simulink model "obwod_naprowadzania_JW"  (Simulink 10.2)
settings: Solver=VariableStepAuto  StartTime=0.0  StopTime=t_sim  MaxStep=0.005  EnableMultiTasking=on
values from neighbouring files (symbols this model uses):
  B_cel0 = deg2rad(-180)    [progaram_symulacyjny.m]
  E_cel0 = deg2rad(0)    [progaram_symulacyjny.m]
  v0 = 300    [progaram_symulacyjny.m]
  x0 = sqrt(23500^2-y0^2-z0^2)+v0*40    [progaram_symulacyjny.m]
  y0 = 0    [progaram_symulacyjny.m]
  z0 = 7000    [progaram_symulacyjny.m]
undefined symbols (not defined in the file or in its folder): beta_0_prim_srcp, caL, epsilon_0_prim_srcp, Fm, Fs, g, h_uwk, Im0, Im1, Is0, Is1, R, RB, RBC, RC, RE, REC, S, tm, ts, tster
libraries: simulink_extras x6, simulink x3
(part 1 of 2)
settings Model: Creator=Marcin  LastModifiedBy=rafal  SimulationMode=accelerator
settings SolverCC: AlgebraicLoopSolver=LineSearch
settings DataIOCC: SaveFormat=Dataset  SignalLoggingSaveFormat=Dataset  SaveOutput=off  SignalLogging=off  DSMLogging=off  SaveTime=off  ReturnWorkspaceOutputs=on  OutputOption=AdditionalOutputTimes  OutputTimes=[0 25]
settings OptimizationCC: BlockReduction=off  BooleanDataType=off  ExpressionDepthLimit=2147483647
settings DebuggingCC: AlgebraicLoopMsg=none  SaveWithParameterizedLinksMsg=none  SignalResolutionControl=TryResolveAllWithWarning  MultiTaskDSMMsg=warning  MultiTaskCondExecSysMsg=none  UnconnectedInputMsg=none  UnconnectedOutputMsg=none  StateNameClashWarn=warning
settings HardwareCC: TargetUnknown=on

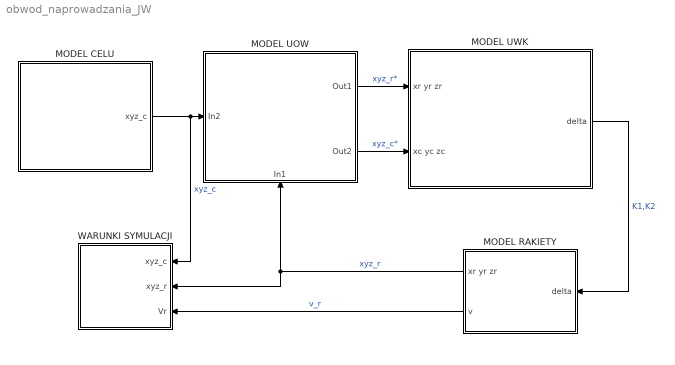
== system obwod_naprowadzania_JW ==
  MODEL CELU : Subsystem
      mask Display: image('C:\Users\rafal\Desktop\project inzynier\MATLAB\APP\photos\photo_target.jpg'); % Use "Edit Image" on toolstrip to change.
  MODEL RAKIETY : Subsystem
      mask Display: image('C:\Users\rafal\Desktop\project inzynier\MATLAB\APP\photos\photo_rocket.jpg'); % Use "Edit Image" on toolstrip to change.
  MODEL UOW : Subsystem
      settings: PortSchema="{\"entries\":[{\"content\":{\"sides\":[{\"content\":{\"connectorIds\":[\"In1\"]},\"type\":\"ConnectorPlacement.EquallySpacedRectSide\",\"uuid\":\"3befb01d-3bbd-4f2b-80c3-c30ac2a777af\"},{\"content\":{\"connectorIds\":[\"Out1\",\"Out2\"],\"side\":\"RIGHT\"},\"type\":\"ConnectorPlacement.EquallySpacedRectSide\",\"uuid\":\"03e5f92e-1691-4957-8f0b-6c1fa9d54603\"},{\"content\":{\"connectorIds\":[],\"side\":\"TOP\"},\"type\":\"ConnectorPlacement.EquallySpacedRectSide\",\"uuid\":\"07804cda-bb58-4fab-8fa4-61420b718606\"},{\"content\":{\"connectorIds\":[\"In2\"],\"side\":\"BOTTOM\"},\"type\":\"ConnectorPlacement.EquallySpacedRectSide\",\"uuid\":\"8550f404-f45b-4210-a410-eab1ae605921\"},{\"content\":{\"connectorIds\":[],\"side\":\"HIDDEN\"},\"type\":\"ConnectorPlacement.EquallySpacedRectSide\",\"uuid\":\"ae5e5650-e780-42f5-87a2-0961b270b42b\"}]},\"type\":\"ConnectorPlacement.EquallySpacedConnector\",\"uuid\":\"f3ed23f3-ebd5-40a8-abbc-f73b2ecd0d2f\"}],\"packageUris\":[\"http://schema.mathworks.com/mf0/Connector/R2020b\"],\"version\":\"1.0\"}"
      mask Display: image('C:\Users\rafal\Desktop\project inzynier\MATLAB\APP\photos\photo_radar.jpg'); % Use "Edit Image" on toolstrip to change.
  MODEL UWK : Subsystem
      mask Display: image('C:\Users\rafal\Desktop\project inzynier\MATLAB\APP\photos\photo_snr.jpg'); % Use "Edit Image" on toolstrip to change.
  WARUNKI SYMULACJI : Subsystem
  wires:
  MODEL UWK/1(delta) -> MODEL RAKIETY/1(delta)  "K1,K2"
  MODEL CELU/1(xyz_c) -> WARUNKI SYMULACJI/1(xyz_c), MODEL UOW/1(In2)  "xyz_c"
  MODEL RAKIETY/1(xr yr zr) -> WARUNKI SYMULACJI/2(xyz_r), MODEL UOW/2(In1)  "xyz_r"
  MODEL UOW/1(Out1) -> MODEL UWK/1(xr yr zr)  "xyz_r*"
  MODEL UOW/2(Out2) -> MODEL UWK/2(xc yc zc)  "xyz_c*"
  MODEL RAKIETY/2(v) -> WARUNKI SYMULACJI/3(Vr)  "v_r"

== system obwod_naprowadzania_JW/MODEL CELU ==
  Bus to Vector1 : BusToVector
  Model samolotu : Subsystem
  Wyliczanie przeciążeń : Subsystem
  Wyliczanie współrzędnych kartezjańskich samolotu : Subsystem
  xyz_c : Outport
  wires:
  Wyliczanie przeciążeń/1(n) -> [n]
  Model samolotu/1(y) -> Wyliczanie przeciążeń/1(In), Wyliczanie współrzędnych kartezjańskich samolotu/1(In)
  [n] -> Model samolotu/1(n)
  Wyliczanie współrzędnych kartezjańskich samolotu/1(xyz_c) -> Bus to Vector1/1
  Bus to Vector1/1 -> xyz_c/1

== system obwod_naprowadzania_JW/MODEL RAKIETY ==
  note: Px
  note: Pz
  note: Py
  note: M
  note: N
  delta : Inport
  10 rownan rozniczkowych : Subsystem
      mask Display: disp('Rownania rakiety')
  Bus Selector : BusSelector  OutputSignals=x_r,y_r,z_r,vr
  Demux : Demux  Outputs=10
      settings: DisplayOption=none
  Demux1 : Demux  Outputs=3
      settings: DisplayOption=none
  Funkcje w rownaniach rozniczkowych : Subsystem
      mask Display: disp('F(t), m(t), Iy(t), Iz(t)')
  Mux : Mux  Inputs=22
  Mux2 : Mux  Inputs=3
  One1 : Constant  OutDataTypeStr=Inherit: Inherit via back propagation
  Timer : Integrator
  To Workspace1 : ToWorkspace  VariableName=r_time  SampleTime=-1
      settings: MaxDataPoints=1
  Zaleznosci miedzy wprowadzonymi ukladami wspolrzednych : Subsystem
      mask Display: disp('mia, beta, alfa')
  Zaleznosci na skladowe sil i momentow aerodynamicznych : Subsystem
      mask Display: disp('Aero')
  "delta 1,2 -> delta m,n" : Subsystem  mask(Delta){}
      mask Display: disp('Delta')
  stala : Constant  Value=-1
  zg(t)*(-1) : Subsystem  mask(Dot Product){}
      mask help:
      | Inner (dot) product.
      | y=sum(u1.*u2)
      mask Help: Computes the inner (dot) product of the inputs: sum(u1.*u2).  The inputs are vectors of the same length. Output is a scalar.
      mask Display: disp('.\n')
  xr yr zr : Outport
  v : Outport  Port=2
  wires:
  Zaleznosci na skladowe sil i momentow aerodynamicznych/1(out_1) -> Mux/18
  Zaleznosci na skladowe sil i momentow aerodynamicznych/2(out_2) -> Mux/19
  Zaleznosci na skladowe sil i momentow aerodynamicznych/3(out_3) -> Mux/20
  Zaleznosci na skladowe sil i momentow aerodynamicznych/4(out_4) -> Mux/21
  Zaleznosci na skladowe sil i momentow aerodynamicznych/5(out_5) -> Mux/22
  Demux/1 -> Mux/1
  Demux/2 -> Mux/2
  Demux/3 -> Mux/3
  Demux/4 -> Mux/4
  Demux/5 -> Mux/5
  Demux/6 -> Mux/6
  Demux/8 -> Mux/8
  Demux/9 -> Mux/9
  Demux/10 -> Mux/10
  Demux/7 -> Mux/7
  Zaleznosci miedzy wprowadzonymi ukladami wspolrzednych/1(out_1) -> Mux/15
  Zaleznosci miedzy wprowadzonymi ukladami wspolrzednych/2(out_2) -> Mux/16, Zaleznosci na skladowe sil i momentow aerodynamicznych/1(beta)
  Zaleznosci miedzy wprowadzonymi ukladami wspolrzednych/3(out_3) -> Mux/17, Zaleznosci na skladowe sil i momentow aerodynamicznych/2(alfa)
  Bus Selector/1 -> Mux2/1  "<x_r>"
  Bus Selector/2 -> Mux2/2  "<y_r>"
  zg(t)*(-1)/1(out_1) -> Mux2/3
  Mux2/1 -> xr yr zr/1
  Demux1/1 -> Mux/11
  Demux1/2 -> Mux/12
  Demux1/3 -> Mux/13, Mux/14
  Funkcje w rownaniach rozniczkowych/1(out_1) -> Demux1/1
  Mux/1 -> 10 rownan rozniczkowych/1(in_1)
  10 rownan rozniczkowych/1(out_1) -> Bus Selector/1, Demux/1, Zaleznosci na skladowe sil i momentow aerodynamicznych/3(1-10), Zaleznosci miedzy wprowadzonymi ukladami wspolrzednych/1(in_1)
  delta/1 -> "delta 1,2 -> delta m,n"/1(delta_1,2)
  "delta 1,2 -> delta m,n"/1(delta_m,n) -> Zaleznosci na skladowe sil i momentow aerodynamicznych/4(delta)
  One1/1 -> Timer/1
  Timer/1 -> To Workspace1/1
  stala/1 -> zg(t)*(-1)/2(in_2)
  Bus Selector/3 -> zg(t)*(-1)/1(in_1)  "<z_r>"
  Bus Selector/4 -> v/1  "<vr>"

== system obwod_naprowadzania_JW/MODEL UOW ==
  In2 : Inport
  In1 : Inport  Port=2
  Cartesian to Spherical : simulink_extras/Transformations/Cartesian to Spherical
      settings: SourceProductBaseCode=SL
  Cartesian to Spherical1 : simulink_extras/Transformations/Cartesian to Spherical
      settings: SourceProductBaseCode=SL
  Demux3 : Demux  Outputs=3
      settings: DisplayOption=none
  Demux4 : Demux  Outputs=3
      settings: DisplayOption=none
  Mux : Mux  Inputs=3
  Mux1 : Mux  Inputs=3
  Spherical to Cartesian : simulink_extras/Transformations/Spherical to Cartesian
      settings: SourceProductBaseCode=SL
  Spherical to Cartesian1 : simulink_extras/Transformations/Spherical to Cartesian
      settings: SourceProductBaseCode=SL
  UOW C : Subsystem
  UOW R : Subsystem
  Out1 : Outport
  Out2 : Outport  Port=2
  wires:
  Demux4/3 -> Cartesian to Spherical/3
  In2/1 -> Demux4/1
  Cartesian to Spherical1/1 -> UOW R/1(R)
  Demux3/2 -> Cartesian to Spherical1/2
  Mux1/1 -> Out1/1
  Demux3/3 -> Cartesian to Spherical1/3
  Cartesian to Spherical/2 -> UOW C/2(B)
  Demux4/1 -> Cartesian to Spherical/1
  Demux3/1 -> Cartesian to Spherical1/1
  Demux4/2 -> Cartesian to Spherical/2
  Cartesian to Spherical/3 -> UOW C/3(E)
  Cartesian to Spherical/1 -> UOW C/1(R)
  Cartesian to Spherical1/2 -> UOW R/2(B)
  Cartesian to Spherical1/3 -> UOW R/3(E)
  In1/1 -> Demux3/1
  Mux/1 -> Out2/1
  UOW R/1(R*) -> Spherical to Cartesian/1
  UOW R/2(B*) -> Spherical to Cartesian/2
  UOW R/3(E*) -> Spherical to Cartesian/3
  Spherical to Cartesian/3 -> Mux1/3
  Spherical to Cartesian/2 -> Mux1/2
  Spherical to Cartesian/1 -> Mux1/1
  UOW C/2(B*) -> Spherical to Cartesian1/2
  UOW C/1(R*) -> Spherical to Cartesian1/1
  UOW C/3(E*) -> Spherical to Cartesian1/3
  Spherical to Cartesian1/3 -> Mux/3
  Spherical to Cartesian1/2 -> Mux/2
  Spherical to Cartesian1/1 -> Mux/1

== system obwod_naprowadzania_JW/MODEL UWK ==
  xr yr zr : Inport
  xc yc zc : Inport  Port=2
  Demux : Demux  Outputs=2
      settings: DisplayOption=none
  Demux1 : Demux  Outputs=2
      settings: DisplayOption=none
  "K -> delta" : Subsystem  mask(Delta){}
      mask Display: disp('Delta')
  Komendy Kierowania Waskie Pasmo : Subsystem  mask(Komendy){}
      mask Display: disp('K1, K2')
  Mux1 : Mux  Inputs=2
  Odchyki : Subsystem  mask(Mask){}
      mask Display: disp('h, fi_prim')
  Przelicznik TP : Subsystem  mask(TP){}
      mask Display: disp('TP')
  delta : Outport
  wires:
  Komendy Kierowania Waskie Pasmo/1(K1) -> "K -> delta"/1(K1)
  Komendy Kierowania Waskie Pasmo/2(K2) -> "K -> delta"/2(K2)
  Przelicznik TP/1(Out) -> Komendy Kierowania Waskie Pasmo/1(In1)
  "K -> delta"/1(delta1) -> Mux1/1
  "K -> delta"/2(delta2) -> Mux1/2
  Demux/1 -> Przelicznik TP/3(fi1c_prim)
  Demux/2 -> Przelicznik TP/4(fi2c_prim)
  Mux1/1 -> delta/1
  Demux1/2 -> Przelicznik TP/2(h2fi2)
  Demux1/1 -> Przelicznik TP/1(h1fi1)
  xr yr zr/1 -> Odchyki/1(xr yr zr)
  xc yc zc/1 -> Odchyki/2(xc yc zc)
  Odchyki/2(fi_prim) -> Demux/1
  Odchyki/1(h) -> Demux1/1
  Odchyki/3(gammaR) -> Komendy Kierowania Waskie Pasmo/2(gammaR)

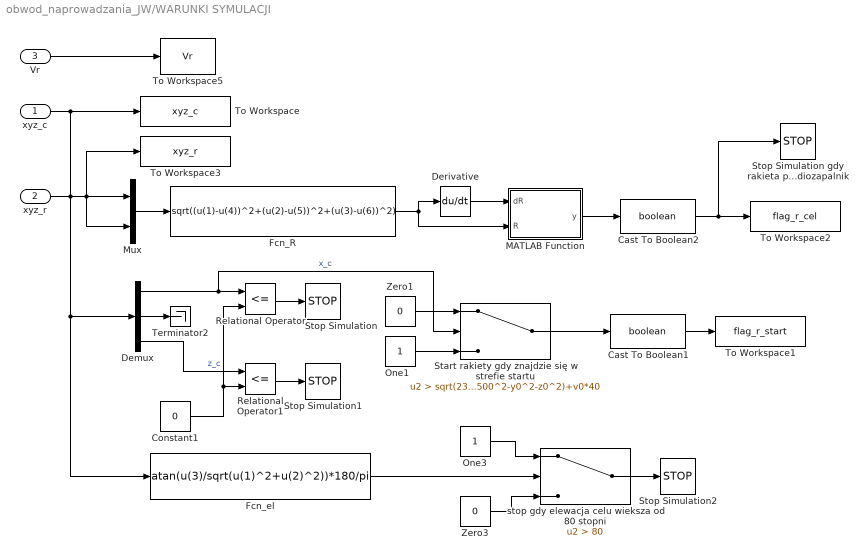
== system obwod_naprowadzania_JW/WARUNKI SYMULACJI ==
  xyz_c : Inport
  xyz_r : Inport  Port=2
  Vr : Inport  Port=3
  Cast To Boolean1 : DataTypeConversion  OutDataTypeStr=boolean
  Cast To Boolean2 : DataTypeConversion  OutDataTypeStr=boolean
  Constant1 : Constant  Value=0
  Demux : Demux  Outputs=3
  Derivative : Derivative
  Fcn_R : Fcn  Expr=sqrt((u(1)-u(4))^2+(u(2)-u(5))^2+(u(3)-u(6))^2)
  Fcn_el : Fcn  Expr=atan(u(3)/sqrt(u(1)^2+u(2)^2))*180/pi
  MATLAB Function : MATLAB Function  TreatAsAtomicUnit=on
  Mux : Mux  Inputs=2
  One1 : Constant  OutDataTypeStr=Inherit: Inherit via back propagation
  One3 : Constant  OutDataTypeStr=Inherit: Inherit via back propagation
  Relational Operator : RelationalOperator  Operator=<=  OutDataTypeStr=boolean  RndMeth=Simplest
  Relational Operator1 : RelationalOperator  Operator=<=  OutDataTypeStr=boolean  RndMeth=Simplest
  Start rakiety gdy znajdzie się w strefie startu : Switch  Criteria=u2 > Threshold  Threshold=sqrt(23500^2-y0^2-z0^2)+v0*40
  Stop Simulation : Stop
  Stop Simulation gdy rakieta przeleci cel lub zadziała radiozapalnik : Stop
  Stop Simulation1 : Stop
  Stop Simulation2 : Stop
  Terminator2 : Terminator
  To Workspace : ToWorkspace  VariableName=xyz_c  SampleTime=0.1
  To Workspace1 : ToWorkspace  VariableName=flag_r_start  SampleTime=-1
  To Workspace2 : ToWorkspace  VariableName=flag_r_cel  SampleTime=-1
  To Workspace3 : ToWorkspace  VariableName=xyz_r  SampleTime=-1
  To Workspace5 : ToWorkspace  VariableName=Vr  SaveFormat=Timeseries  SampleTime=0.01
  Zero1 : Constant  Value=0  OutDataTypeStr=Inherit: Inherit via back propagation
  Zero3 : Constant  Value=0  OutDataTypeStr=Inherit: Inherit via back propagation
  "stop gdy elewacja celu wieksza od 80 stopni " : Switch  Criteria=u2 > Threshold  Threshold=80
  wires:
  Zero1/1 -> Start rakiety gdy znajdzie się w strefie startu/1
  Cast To Boolean1/1 -> To Workspace1/1
  Start rakiety gdy znajdzie się w strefie startu/1 -> Cast To Boolean1/1
  Mux/1 -> Fcn_R/1
  One1/1 -> Start rakiety gdy znajdzie się w strefie startu/3
  Demux/2 -> Terminator2/1
  Constant1/1 -> Relational Operator1/2, Relational Operator/2
  Demux/3 -> Relational Operator1/1  "z_c"
  Relational Operator1/1 -> Stop Simulation1/1
  Demux/1 -> Start rakiety gdy znajdzie się w strefie startu/2, Relational Operator/1  "x_c"
  Relational Operator/1 -> Stop Simulation/1
  Fcn_el/1 -> "stop gdy elewacja celu wieksza od 80 stopni "/2
  "stop gdy elewacja celu wieksza od 80 stopni "/1 -> Stop Simulation2/1
  One3/1 -> "stop gdy elewacja celu wieksza od 80 stopni "/1
  Zero3/1 -> "stop gdy elewacja celu wieksza od 80 stopni "/3
  Fcn_R/1 -> MATLAB Function/2(R), Derivative/1
  Derivative/1 -> MATLAB Function/1(dR)
  MATLAB Function/1(y) -> Cast To Boolean2/1
  Cast To Boolean2/1 -> Stop Simulation gdy rakieta przeleci cel lub zadziała radiozapalnik/1, To Workspace2/1
  xyz_c/1 -> Fcn_el/1, Demux/1, Mux/1, To Workspace/1
  xyz_r/1 -> Mux/2, To Workspace3/1
  Vr/1 -> To Workspace5/1

== system obwod_naprowadzania_JW/MODEL CELU/Model samolotu ==
  note: Układ współrzędny związany z samolotem
  note: oś wektora v
  note: elewacja
  note: azymut
  n : Inport
  Delay : Delay  DelayLength=1
  Gain1 : Gain  Gain=-1
  Gain4 : Gain  Gain=180/pi
  Gain5 : Gain  Gain=180/pi
  Integrator : Integrator  InitialCondition=v0
  Integrator3 : Integrator  InitialCondition=B_cel0
  Integrator8 : Integrator  InitialCondition=E_cel0
  Macierz sterowania przyrostem kąta w azymucie samolotu : FromWorkspace  VariableName=[T B_cel_dot]
  Macierz sterowania przyrostem kąta w elewacji samolotu : FromWorkspace  VariableName=[T E_cel_dot]
  "Macierz sterowania przyrostem prędkości samolotu " : FromWorkspace  VariableName=[T Ac]
  Ogranicznik przeciążenia  wypadkowego (max 9g) : Subsystem
  Ogranicznik przeciążenia azymut (max 4g) : Subsystem
  Ogranicznik przeciążenia elewacja (max 8g) : Subsystem
  Scope2 : Scope  NumInputPorts=2
  To Workspace1 : ToWorkspace  VariableName=Vc  SaveFormat=Timeseries  SampleTime=0.25
  Out Bus Element : Outport  PortName=y  Element=v_c
  Out Bus Element1 : Outport  PortName=y  Element=a_c
  Out Bus Element2 : Outport  PortName=y  Element=B_cel
  Out Bus Element3 : Outport  PortName=y  Element=E_cel
  wires:
  Macierz sterowania przyrostem kąta w azymucie samolotu/1 -> Ogranicznik przeciążenia azymut (max 4g)/1(u)
  Ogranicznik przeciążenia elewacja (max 8g)/1(y) -> Gain5/1, Integrator8/1  "E_cel dot"
  Integrator/1 -> To Workspace1/1, Out Bus Element/1, [v]  "v_c"
  Macierz sterowania przyrostem kąta w elewacji samolotu/1 -> Ogranicznik przeciążenia elewacja (max 8g)/1(u), Gain4/1
  Ogranicznik przeciążenia  wypadkowego (max 9g)/1(y) -> Out Bus Element1/1, Integrator/1  "a_c"
  [v] -> Ogranicznik przeciążenia elewacja (max 8g)/2(v)
  Ogranicznik przeciążenia azymut (max 4g)/1(y) -> Gain1/1
  [v] -> Ogranicznik przeciążenia azymut (max 4g)/2(v)
  Gain1/1 -> Integrator3/1  "B_cel dot"
  "Macierz sterowania przyrostem prędkości samolotu "/1 -> Ogranicznik przeciążenia  wypadkowego (max 9g)/1(u)  "u"
  Integrator3/1 -> Out Bus Element2/1  "B_cel"
  Integrator8/1 -> Out Bus Element3/1  "E_cel"
  Gain4/1 -> Scope2/1  "u"
  Gain5/1 -> Scope2/2  "y"
  n/1 -> Delay/1
  Delay/1 -> Ogranicznik przeciążenia  wypadkowego (max 9g)/2(n)

== system obwod_naprowadzania_JW/MODEL CELU/Wyliczanie przeciążeń ==
  In : Inport
  Bus Selector1 : BusSelector  OutputSignals=a_c,v_c,B_cel,E_cel
  Derivative1 : Derivative
  Derivative2 : Derivative
  Gain : Gain  Gain=1/9.81
  IC : InitialCondition  Value=0
  Mux3 : Mux  Inputs=3
  Mux5 : Mux  Inputs=3
  Scope : Scope  NumInputPorts=2
  przeciazenie wypadkowe : Fcn  Expr=sqrt(u(1)^2+u(2)^2+u(3)^2)
  przeciazenie_azy : Fcn  Expr=u(1)*u(2)/9.81
  przeciazenie_el : Fcn  Expr=u(1)*u(3)/9.81
  n : Outport
  wires:
  Derivative2/1 -> Mux3/3  "u(3)"
  Mux3/1 -> przeciazenie_azy/1, przeciazenie_el/1
  przeciazenie wypadkowe/1 -> Scope/2  "n"
  przeciazenie_azy/1 -> Mux5/2  "n_B"
  przeciazenie_el/1 -> Mux5/3  "n_E"
  Bus Selector1/4 -> Derivative2/1  "<E_cel>"
  Gain/1 -> Mux5/1  "n_s"
  Bus Selector1/3 -> Derivative1/1  "<B_cel>"
  Bus Selector1/2 -> Mux3/1  "<v_c>"
  Derivative1/1 -> Mux3/2  "u(2)"
  In/1 -> Bus Selector1/1
  Bus Selector1/1 -> Gain/1  "<a_c>"
  Mux5/1 -> IC/1, Scope/1, przeciazenie wypadkowe/1
  IC/1 -> n/1

== system obwod_naprowadzania_JW/MODEL CELU/Wyliczanie współrzędnych kartezjańskich samolotu ==
  note: Kartezjański układ współrzędnych xyz
  In : Inport
  Bus Creator : BusCreator  Inputs=3
  Bus Selector : BusSelector  OutputSignals=v_c,B_cel,E_cel
  Integrator4 : Integrator  InitialCondition=x0
  Integrator5 : Integrator  InitialCondition=y0
  Integrator6 : Integrator  InitialCondition=z0
  Mux : Mux  Inputs=3
  Mux1 : Mux  Inputs=3
  Scope2 : Scope
  modul : Fcn  Expr=sqrt(u(1)^2+u(2)^2+u(3)^2)
  vx : Fcn  Expr=u(1)*cos(u(2))*cos(u(3))
  vy : Fcn  Expr=u(1)*sin(u(2))*cos(u(3))
  vz : Fcn  Expr=u(1)*sin(u(3))
  xyz_c : Outport
  wires:
  vy/1 -> Integrator5/1, Mux1/2  "vy"
  Mux1/1 -> modul/1
  vz/1 -> Mux1/3, Integrator6/1  "vz"
  modul/1 -> Scope2/1  "modul_predkosci"
  vx/1 -> Mux1/1, Integrator4/1  "vx"
  Bus Creator/1 -> xyz_c/1
  Integrator6/1 -> Bus Creator/3  "z_c"
  Integrator5/1 -> Bus Creator/2  "y_c"
  Integrator4/1 -> Bus Creator/1  "x_c"
  In/1 -> Bus Selector/1
  Mux/1 -> vz/1, vy/1, vx/1
  Bus Selector/1 -> Mux/1  "<v_c>"
  Bus Selector/2 -> Mux/2  "<B_cel>"
  Bus Selector/3 -> Mux/3  "<E_cel>"

== system obwod_naprowadzania_JW/MODEL RAKIETY/10 rownan rozniczkowych ==
  in_1 : Inport
  Bus Creator : BusCreator  Inputs=10
  Sub1 : Subsystem
      mask Display: disp('V')
  Sub10 : Subsystem
      mask Display: disp('psi')
  Sub2 : Subsystem
      mask Display: disp('kappa')
  Sub3 : Subsystem
      mask Display: disp('gamma')
  Sub4 : Subsystem
      mask Display: disp('xg')
  Sub5 : Subsystem
      mask Display: disp('yg')
  Sub6 : Subsystem
      mask Display: disp('zg')
  Sub7 : Subsystem
      mask Display: disp('q')
  Sub8 : Subsystem
      mask Display: disp('r')
  Sub9 : Subsystem
      mask Display: disp('theta')
  out_1 : Outport
  wires:
  Sub1/1(out_1) -> Bus Creator/1  "vr"
  Sub2/1(out_1) -> Bus Creator/2
  Sub3/1(out_1) -> Bus Creator/3
  Sub10/1(out_1) -> Bus Creator/10
  Sub9/1(out_1) -> Bus Creator/9
  Sub8/1(out_1) -> Bus Creator/8
  Sub7/1(out_1) -> Bus Creator/7
  Sub6/1(out_1) -> Bus Creator/6  "z_r"
  Sub5/1(out_1) -> Bus Creator/5  "y_r"
  Sub4/1(out_1) -> Bus Creator/4  "x_r"
  Bus Creator/1 -> out_1/1
  in_1/1 -> Sub1/1(in_1), Sub2/1(in_1), Sub3/1(in_1), Sub4/1(in_1), Sub5/1(in_1), Sub6/1(in_1), Sub7/1(in_1), Sub8/1(in_1), Sub9/1(in_1), Sub10/1(in_1)

== system obwod_naprowadzania_JW/MODEL RAKIETY/Funkcje w rownaniach rozniczkowych ==
  F(t) : Subsystem
      mask Display: disp('F(t)')
  Iy(t) Iz(t) : Subsystem
      mask Display: disp('I(t)')
  Mux2 : Mux  Inputs=3
  czas : Clock
  m(t) : Subsystem
      mask Display: disp('m(t)')
  out_1 : Outport
  wires:
  czas/1 -> F(t)/1(in_1), m(t)/1(in_1), Iy(t) Iz(t)/1(in_1)
  F(t)/1(out_1) -> Mux2/1
  m(t)/1(out_1) -> Mux2/2
  Iy(t) Iz(t)/1(out_1) -> Mux2/3
  Mux2/1 -> out_1/1

== system obwod_naprowadzania_JW/MODEL RAKIETY/Zaleznosci miedzy wprowadzonymi ukladami wspolrzednych ==
  in_1 : Inport
  alfa : Fcn  Expr=(1/cos(asin(cos(u[3])*cos(fi)*sin(u[2]-u[10])+sin(fi)*sin(u[9])*cos(u[3])*cos(u[2]-u[10])-sin(u[3])*cos(u[9])*sin(fi))))*(cos(fi)*sin(u[9])*cos(u[3])*cos(u[2]-u[10])-cos(u[3])*sin(fi)*sin(u[2]-u[10])-sin(u[3])*cos(fi)*cos(u[9]))
  beta : Fcn  Expr=asin(cos(u[3])*cos(fi)*sin(u[2]-u[10])+sin(fi)*sin(u[9])*cos(u[3])*cos(u[2]-u[10])-sin(u[3])*cos(u[9])*sin(fi))
  mia : Fcn  Expr=(1/cos(asin(cos(u[3])*cos(fi)*sin(u[2]-u[10])+sin(fi)*sin(u[9])*cos(u[3])*cos(u[2]-u[10])-sin(u[3])*cos(u[9])*sin(fi))))*(sin(u[3])*cos(fi)*sin(u[2]-u[10])+sin(fi)*sin(u[9])*sin(u[3])*cos(u[2]-u[10])+sin(fi)*cos(u[9])*cos(u[3]))
  out_1 : Outport
  out_2 : Outport  Port=2
  out_3 : Outport  Port=3
  wires:
  in_1/1 -> beta/1, alfa/1, mia/1
  mia/1 -> out_1/1
  alfa/1 -> out_3/1
  beta/1 -> out_2/1

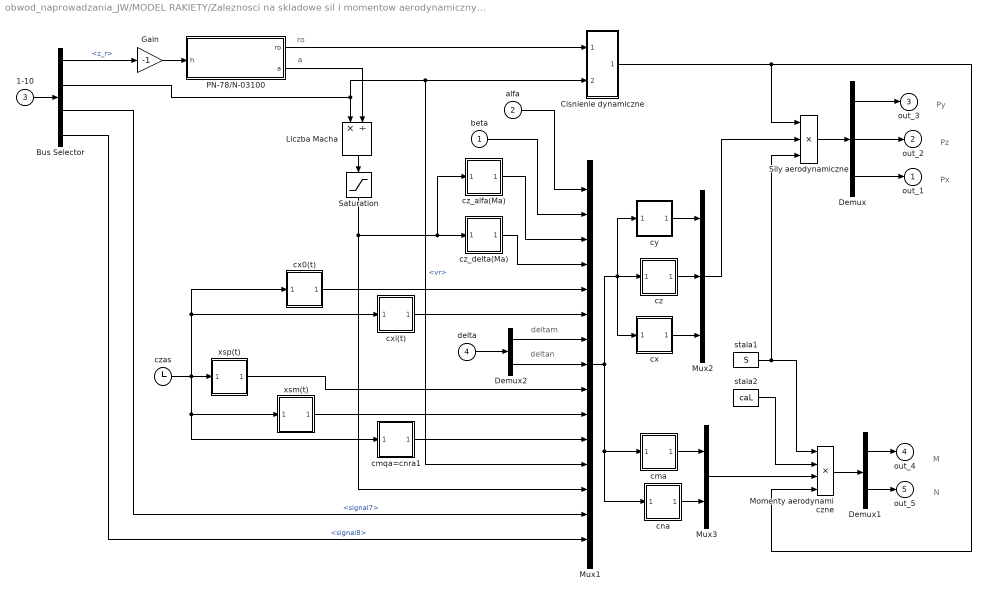
== system obwod_naprowadzania_JW/MODEL RAKIETY/Zaleznosci na skladowe sil i momentow aerodynamicznych ==
  note: Py
  note: Pz
  note: N
  note: M
  note: Px
  note: deltam
  note: deltan
  note: ro
  note: a
  beta : Inport
  alfa : Inport  Port=2
  1-10 : Inport  Port=3
  delta : Inport  Port=4
  Bus Selector : BusSelector  OutputSignals=z_r,vr,signal7,signal8
  Cisnienie dynamiczne : Subsystem
      mask Display: disp('q_dyn')
  Demux : Demux  Outputs=3
      settings: DisplayOption=none
  Demux1 : Demux  Outputs=2
      settings: DisplayOption=none
  Demux2 : Demux  Outputs=2
      settings: DisplayOption=none
  Gain : Gain  Gain=-1  SaturateOnIntegerOverflow=on  OutDataTypeStr=Inherit: Same as input  ParamDataTypeStr=Inherit: Same as input
  Liczba Macha : Product  Inputs=*/  InputSameDT=on  RndMeth=Zero  SaturateOnIntegerOverflow=on  OutDataTypeStr=Inherit: Same as first input
  Momenty aerodynamiczne : Product  Inputs=4  InputSameDT=on  RndMeth=Zero  SaturateOnIntegerOverflow=on  OutDataTypeStr=Inherit: Same as first input
  Mux1 : Mux  Inputs=15
  Mux2 : Mux  Inputs=3
  Mux3 : Mux  Inputs=2
  "PN-78/N-03100  " : Subsystem
      mask Display: disp('Atmosfera wzorcowa')
  Saturation : Saturate  UpperLimit=2.8  LowerLimit=1.2
  Sily aerodynamiczne : Product  Inputs=3  InputSameDT=on  RndMeth=Zero  SaturateOnIntegerOverflow=on  OutDataTypeStr=Inherit: Same as first input
  cma : Subsystem
  cmqa=cnra1 : Subsystem
  cna : Subsystem
  cx : Subsystem
  cx0(t) : Subsystem
  cxi(t) : Subsystem
  cy : Subsystem
  cz : Subsystem
  cz_alfa(Ma) : Subsystem
  cz_delta(Ma) : Subsystem
  czas : Clock
  stala1 : Constant  Value=S
  stala2 : Constant  Value=caL
  xsm(t) : Subsystem
  xsp(t) : Subsystem
  out_1 : Outport
  out_2 : Outport  Port=2
  out_3 : Outport  Port=3
  out_4 : Outport  Port=4
  out_5 : Outport  Port=5
  wires:
  "PN-78/N-03100  "/1(ro) -> Cisnienie dynamiczne/1(In1)
  1-10/1 -> Bus Selector/1
  cz_alfa(Ma)/1(out_1) -> Mux1/3
  cz_delta(Ma)/1(out_1) -> Mux1/4
  cxi(t)/1(out_1) -> Mux1/6
  Cisnienie dynamiczne/1(Out1) -> Momenty aerodynamiczne/4, Sily aerodynamiczne/1
  alfa/1 -> Mux1/1
  beta/1 -> Mux1/2
  Mux1/1 -> cx/1(in_1), cz/1(in_1), cy/1(in_1), cma/1(in_1), cna/1(in_1)
  cy/1(out_1) -> Mux2/1
  cz/1(out_1) -> Mux2/2
  cx/1(out_1) -> Mux2/3
  Sily aerodynamiczne/1 -> Demux/1
  Demux/3 -> out_1/1
  Demux/2 -> out_2/1
  Demux/1 -> out_3/1
  xsp(t)/1(out_1) -> Mux1/9
  xsm(t)/1(out_1) -> Mux1/10
  cmqa=cnra1/1(out_1) -> Mux1/11
  Bus Selector/3 -> Mux1/14  "<signal7>"
  Bus Selector/4 -> Mux1/15  "<signal8>"
  cma/1(out_1) -> Mux3/1
  cna/1(out_1) -> Mux3/2
  Demux1/1 -> out_4/1
  Demux1/2 -> out_5/1
  Demux2/1 -> Mux1/7
  Demux2/2 -> Mux1/8
  delta/1 -> Demux2/1
  Mux2/1 -> Sily aerodynamiczne/2
  stala1/1 -> Sily aerodynamiczne/3, Momenty aerodynamiczne/1
  stala2/1 -> Momenty aerodynamiczne/2
  Mux3/1 -> Momenty aerodynamiczne/3
  Momenty aerodynamiczne/1 -> Demux1/1
  Bus Selector/1 -> Gain/1  "<z_r>"
  Gain/1 -> "PN-78/N-03100  "/1(h)
  cx0(t)/1(out_1) -> Mux1/5
  czas/1 -> xsp(t)/1(in_1), xsm(t)/1(in_1), cmqa=cnra1/1(in_1), cxi(t)/1(in_1), cx0(t)/1(in_1)
  Bus Selector/2 -> Cisnienie dynamiczne/2(In2), Mux1/12, Liczba Macha/1  "<vr>"
  "PN-78/N-03100  "/2(a) -> Liczba Macha/2
  Liczba Macha/1 -> Saturation/1
  Saturation/1 -> Mux1/13, cz_delta(Ma)/1(in_1), cz_alfa(Ma)/1(in_1)

== system obwod_naprowadzania_JW/MODEL RAKIETY/delta 1,2 -> delta m,n ==
  delta_1,2 : Inport
  Constant : Constant  Value=sqrt(2)
  Demux : Demux  Outputs=2
      settings: DisplayOption=none
  Mux : Mux  Inputs=2
  Product : Product  Inputs=*/  InputSameDT=on  RndMeth=Zero  SaturateOnIntegerOverflow=on  OutDataTypeStr=Inherit: Same as first input
  Sum1 : Sum  InputSameDT=on  SaturateOnIntegerOverflow=on  OutDataTypeStr=Inherit: Same as first input
  Sum5 : Sum  Inputs=+-  InputSameDT=on  SaturateOnIntegerOverflow=on  OutDataTypeStr=Inherit: Same as first input
  delta_m,n : Outport
  wires:
  delta_1,2/1 -> Demux/1
  Demux/1 -> Sum5/1, Sum1/1
  Demux/2 -> Sum5/2, Sum1/2
  Constant/1 -> Product/2
  Sum5/1 -> Mux/1
  Sum1/1 -> Mux/2
  Mux/1 -> Product/1
  Product/1 -> delta_m,n/1

== system obwod_naprowadzania_JW/MODEL RAKIETY/zg(t)*(-1) ==
  in_1 : Inport
  in_2 : Inport  Port=2
  Product : Product  InputSameDT=on  RndMeth=Zero  SaturateOnIntegerOverflow=on  OutDataTypeStr=Inherit: Same as first input
  Sum : Sum  Inputs=+  InputSameDT=on  SaturateOnIntegerOverflow=on  OutDataTypeStr=Inherit: Same as first input
  out_1 : Outport
  wires:
  in_2/1 -> Product/2
  in_1/1 -> Product/1
  Product/1 -> Sum/1
  Sum/1 -> out_1/1

== system obwod_naprowadzania_JW/MODEL UOW/UOW C ==
  R : Inport
  B : Inport  Port=2
  E : Inport  Port=3
  Constant : Constant  Value=RBC
  Constant1 : Constant  Value=REC
  Constant2 : Constant  Value=RC
  Gain : Gain  Gain=pi/180
  Gain2 : Gain  Gain=pi/180
  Sum : Sum  Inputs=|++
  Sum1 : Sum  Inputs=++|
  Sum2 : Sum  Inputs=++|
  R* : Outport
  B* : Outport  Port=2
  E* : Outport  Port=3
  wires:
  Constant/1 -> Gain/1
  B/1 -> Sum/1
  Gain/1 -> Sum/2
  Sum/1 -> B*/1
  Sum1/1 -> E*/1
  E/1 -> Sum1/2
  Gain2/1 -> Sum1/1
  Constant1/1 -> Gain2/1
  Constant2/1 -> Sum2/1
  R/1 -> Sum2/2
  Sum2/1 -> R*/1

== system obwod_naprowadzania_JW/MODEL UOW/UOW R ==
  R : Inport
  B : Inport  Port=2
  E : Inport  Port=3
  Constant : Constant  Value=RB
  Constant1 : Constant  Value=RE
  Constant2 : Constant  Value=R
  Gain : Gain  Gain=pi/180
  Gain2 : Gain  Gain=pi/180
  Sum : Sum  Inputs=|++
  Sum1 : Sum  Inputs=++|
  Sum2 : Sum  Inputs=++|
  R* : Outport
  B* : Outport  Port=2
  E* : Outport  Port=3
  wires:
  Constant/1 -> Gain/1
  B/1 -> Sum/1
  Gain/1 -> Sum/2
  Sum/1 -> B*/1
  Sum1/1 -> E*/1
  E/1 -> Sum1/2
  Gain2/1 -> Sum1/1
  Constant1/1 -> Gain2/1
  R/1 -> Sum2/2
  Sum2/1 -> R*/1
  Constant2/1 -> Sum2/1

== system obwod_naprowadzania_JW/MODEL UWK/K -> delta ==
  K1 : Inport
  K2 : Inport  Port=2
  Constant : Constant  Value=-0.0067
  Demux : Demux  Outputs=2
      settings: DisplayOption=none
  Mux : Mux  Inputs=2
  Product : Product  InputSameDT=on  RndMeth=Zero  SaturateOnIntegerOverflow=on  OutDataTypeStr=Inherit: Same as first input
  Saturation : Saturate  UpperLimit=26*pi/180  LowerLimit=-26*pi/180
  delta1 : Outport
  delta2 : Outport  Port=2
  wires:
  K1/1 -> Mux/1
  K2/1 -> Mux/2
  Mux/1 -> Product/1
  Constant/1 -> Product/2
  Product/1 -> Saturation/1
  Saturation/1 -> Demux/1
  Demux/1 -> delta1/1
  Demux/2 -> delta2/1

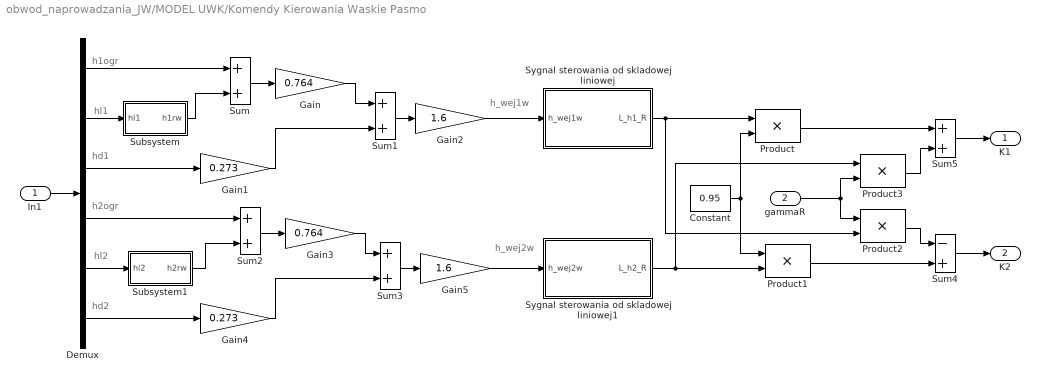
== system obwod_naprowadzania_JW/MODEL UWK/Komendy Kierowania Waskie Pasmo ==
  note: h_wej1w
  note: h_wej2w
  note: h1ogr
  note: hl1
  note: hd1
  note: h2ogr
  note: hl2
  note: hd2
  In1 : Inport
  gammaR : Inport  Port=2
  Constant : Constant  Value=0.95
  Demux : Demux  Outputs=6
      settings: DisplayOption=none
  Gain : Gain  Gain=0.764  SaturateOnIntegerOverflow=on  OutDataTypeStr=Inherit: Same as input  ParamDataTypeStr=Inherit: Same as input
  Gain1 : Gain  Gain=0.273  SaturateOnIntegerOverflow=on  OutDataTypeStr=Inherit: Same as input  ParamDataTypeStr=Inherit: Same as input
  Gain2 : Gain  Gain=1.6  SaturateOnIntegerOverflow=on  OutDataTypeStr=Inherit: Same as input  ParamDataTypeStr=Inherit: Same as input
  Gain3 : Gain  Gain=0.764  SaturateOnIntegerOverflow=on  OutDataTypeStr=Inherit: Same as input  ParamDataTypeStr=Inherit: Same as input
  Gain4 : Gain  Gain=0.273  SaturateOnIntegerOverflow=on  OutDataTypeStr=Inherit: Same as input  ParamDataTypeStr=Inherit: Same as input
  Gain5 : Gain  Gain=1.6  SaturateOnIntegerOverflow=on  OutDataTypeStr=Inherit: Same as input  ParamDataTypeStr=Inherit: Same as input
  Product{,1..3} (4 alike) : Product  InputSameDT=on  RndMeth=Zero  SaturateOnIntegerOverflow=on  OutDataTypeStr=Inherit: Same as first input
  Subsystem : Subsystem
  Subsystem1 : Subsystem
  Sum{,1..3,5} (5 alike) : Sum  InputSameDT=on  SaturateOnIntegerOverflow=on  OutDataTypeStr=Inherit: Same as first input
  Sum4 : Sum  Inputs=-+  InputSameDT=on  SaturateOnIntegerOverflow=on  OutDataTypeStr=Inherit: Same as first input
  Sygnal sterowania od skladowej liniowej : Subsystem
  Sygnal sterowania od skladowej liniowej1 : Subsystem
  K1 : Outport
  K2 : Outport  Port=2
  wires:
  Demux/2 -> Subsystem/1(hl1)
  Demux/1 -> Sum/1
  Subsystem/1(h1rw) -> Sum/2
  Sum/1 -> Gain/1
  Gain/1 -> Sum1/1
  Gain1/1 -> Sum1/2
  Sum1/1 -> Gain2/1
  Gain2/1 -> Sygnal sterowania od skladowej liniowej/1(h_wej1w)
  Subsystem1/1(h2rw) -> Sum2/2
  Sum2/1 -> Gain3/1
  Gain3/1 -> Sum3/1
  Gain4/1 -> Sum3/2
  Sum3/1 -> Gain5/1
  Gain5/1 -> Sygnal sterowania od skladowej liniowej1/1(h_wej2w)
  Demux/3 -> Gain1/1
  Demux/5 -> Subsystem1/1(hl2)
  Demux/4 -> Sum2/1
  Demux/6 -> Gain4/1
  In1/1 -> Demux/1
  Sygnal sterowania od skladowej liniowej/1(L_h1_R) -> Product2/2, Product/1
  Constant/1 -> Product/2, Product1/1
  Sygnal sterowania od skladowej liniowej1/1(L_h2_R) -> Product3/1, Product1/2
  Product/1 -> Sum5/1
  Product3/1 -> Sum5/2
  Sum5/1 -> K1/1
  Product2/1 -> Sum4/1
  Product1/1 -> Sum4/2
  Sum4/1 -> K2/1
  gammaR/1 -> Product2/1, Product3/2

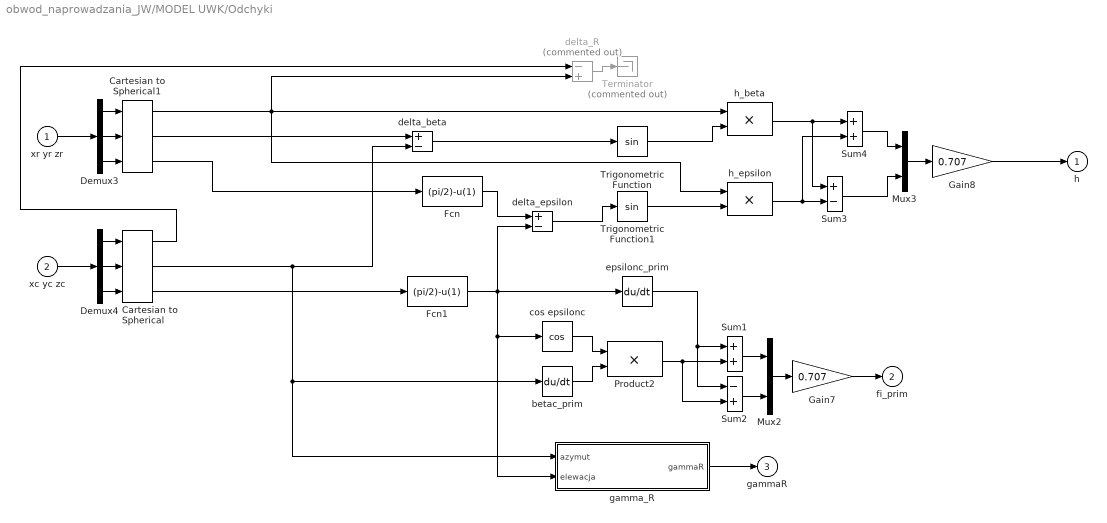
== system obwod_naprowadzania_JW/MODEL UWK/Odchyki ==
  xr yr zr : Inport
  xc yc zc : Inport  Port=2
  Cartesian to Spherical : simulink_extras/Transformations/Cartesian to Spherical
      settings: SourceProductBaseCode=SL
  Cartesian to Spherical1 : simulink_extras/Transformations/Cartesian to Spherical
      settings: SourceProductBaseCode=SL
  Demux3 : Demux  Outputs=3
      settings: DisplayOption=none
  Demux4 : Demux  Outputs=3
      settings: DisplayOption=none
  Fcn : Fcn  Expr=(pi/2)-u(1)
  Fcn1 : Fcn  Expr=(pi/2)-u(1)
  Gain7 : Gain  Gain=0.707  SaturateOnIntegerOverflow=on  OutDataTypeStr=Inherit: Same as input  ParamDataTypeStr=Inherit: Same as input
  Gain8 : Gain  Gain=0.707  SaturateOnIntegerOverflow=on  OutDataTypeStr=Inherit: Same as input  ParamDataTypeStr=Inherit: Same as input
  Mux2 : Mux  Inputs=2
  Mux3 : Mux  Inputs=2
  Product2 : Product  InputSameDT=on  RndMeth=Zero  SaturateOnIntegerOverflow=on  OutDataTypeStr=Inherit: Same as first input
  Sum1 : Sum  InputSameDT=on  SaturateOnIntegerOverflow=on  OutDataTypeStr=Inherit: Same as first input
  Sum2 : Sum  Inputs=-+  InputSameDT=on  SaturateOnIntegerOverflow=on  OutDataTypeStr=Inherit: Same as first input
  Sum3 : Sum  Inputs=+-  InputSameDT=on  SaturateOnIntegerOverflow=on  OutDataTypeStr=Inherit: Same as first input
  Sum4 : Sum  InputSameDT=on  SaturateOnIntegerOverflow=on  OutDataTypeStr=Inherit: Same as first input
  Terminator : Terminator  Commented=on
  Trigonometric Function : Trigonometry
  Trigonometric Function1 : Trigonometry
  betac_prim : Derivative
  cos epsilonc : Trigonometry  Operator=cos
  delta_R : Sum  Commented=on  Inputs=-+  InputSameDT=on  SaturateOnIntegerOverflow=on  OutDataTypeStr=Inherit: Same as first input
  delta_beta : Sum  Inputs=+-  InputSameDT=on  SaturateOnIntegerOverflow=on  OutDataTypeStr=Inherit: Same as first input
  delta_epsilon : Sum  Inputs=+-  InputSameDT=on  SaturateOnIntegerOverflow=on  OutDataTypeStr=Inherit: Same as first input
  epsilonc_prim : Derivative
  gamma_R : Subsystem  mask(Delta){}
      mask Display: disp('Kat wichrowania')
  h_beta : Product  InputSameDT=on  RndMeth=Zero  SaturateOnIntegerOverflow=on  OutDataTypeStr=Inherit: Same as first input
  h_epsilon : Product  InputSameDT=on  RndMeth=Zero  SaturateOnIntegerOverflow=on  OutDataTypeStr=Inherit: Same as first input
  h : Outport
  fi_prim : Outport  Port=2
  gammaR : Outport  Port=3
  wires:
  delta_epsilon/1 -> Trigonometric Function1/1
  h_beta/1 -> Sum3/1, Sum4/1
  h_epsilon/1 -> Sum3/2, Sum4/2
  Sum1/1 -> Mux2/1
  Sum2/1 -> Mux2/2
  Mux2/1 -> Gain7/1
  Mux3/1 -> Gain8/1
  Sum3/1 -> Mux3/2
  Sum4/1 -> Mux3/1
  xr yr zr/1 -> Demux3/1
  Demux3/1 -> Cartesian to Spherical1/1
  Demux3/2 -> Cartesian to Spherical1/2
  Demux3/3 -> Cartesian to Spherical1/3
  Demux4/1 -> Cartesian to Spherical/1
  Demux4/2 -> Cartesian to Spherical/2
  Demux4/3 -> Cartesian to Spherical/3
  xc yc zc/1 -> Demux4/1
  Fcn/1 -> delta_epsilon/1
  Fcn1/1 -> epsilonc_prim/1, cos epsilonc/1, gamma_R/2(elewacja), delta_epsilon/2
  delta_beta/1 -> Trigonometric Function/1
  Trigonometric Function/1 -> h_beta/2
  Trigonometric Function1/1 -> h_epsilon/2
  Gain8/1 -> h/1
  cos epsilonc/1 -> Product2/1
  betac_prim/1 -> Product2/2
  Product2/1 -> Sum1/2, Sum2/2
  epsilonc_prim/1 -> Sum2/1, Sum1/1
  Gain7/1 -> fi_prim/1
  gamma_R/1(gammaR) -> gammaR/1
  Cartesian to Spherical/2 -> gamma_R/1(azymut), betac_prim/1, delta_beta/2
  Cartesian to Spherical/3 -> Fcn1/1
  Cartesian to Spherical/1 -> delta_R/1
  delta_R/1 -> Terminator/1
  Cartesian to Spherical1/1 -> h_epsilon/1, delta_R/2, h_beta/1
  Cartesian to Spherical1/2 -> delta_beta/1
  Cartesian to Spherical1/3 -> Fcn/1

== system obwod_naprowadzania_JW/MODEL UWK/Przelicznik TP ==
  note: h1ogr
  note: hl1
  note: hd1
  note: h2ogr
  note: hl2
  note: hd2
  h1fi1 : Inport
  h2fi2 : Inport  Port=2
  fi1c_prim : Inport  Port=3
  fi2c_prim : Inport  Port=4
  Constant : Constant  Value=-916.8
  Constant1 : Constant  Value=3.5
  Demux : Demux  Outputs=2
      settings: DisplayOption=none
  Mux1 : Mux  Inputs=6
  Mux2 : Mux  Inputs=2
  Product : Product  InputSameDT=on  RndMeth=Zero  SaturateOnIntegerOverflow=on  OutDataTypeStr=Inherit: Same as first input
  Sum : Sum  Inputs=+-  InputSameDT=on  SaturateOnIntegerOverflow=on  OutDataTypeStr=Inherit: Same as first input
  Sum1 : Sum  InputSameDT=on  SaturateOnIntegerOverflow=on  OutDataTypeStr=Inherit: Same as first input
  Out : Outport
  wires:
  Mux1/1 -> Out/1
  fi1c_prim/1 -> Mux2/1
  fi2c_prim/1 -> Mux2/2
  Mux2/1 -> Product/1
  Constant/1 -> Product/2
  Product/1 -> Demux/1
  Demux/1 -> Sum/1
  Constant1/1 -> Sum/2, Sum1/2
  Demux/2 -> Sum1/1
  Sum/1 -> Mux1/3
  Sum1/1 -> Mux1/6
  h1fi1/1 -> Mux1/2, Mux1/1
  h2fi2/1 -> Mux1/5, Mux1/4

== system obwod_naprowadzania_JW/MODEL CELU/Model samolotu/Ogranicznik przeciążenia  wypadkowego (max 9g) ==
  u : Inport
  n : Inport  Port=2
  Fcn : Fcn  Expr=sqrt(abs(9^2-u(3)^2-u(2)^2))*9.81
  Fcn2 : Fcn  Expr=sqrt(abs(9^2-u(3)^2-u(2)^2))*-9.81
  IC : InitialCondition  Value=0
  Saturation Dynamic : simulink/Discontinuities/Saturation Dynamic  OutMin=[]  OutMax=[]  OutDataTypeStr=Inherit: Same as second input  OutDataType=fixdt(1, 16)  OutScaling=2^-10  DoSatur=off
  Sum : Sum  Inputs=|++
  sprzężenie zwrotne (wzrost prędkości o zadaną wartość) : Subsystem
  y : Outport
  wires:
  n/1 -> Fcn2/1, Fcn/1
  Fcn2/1 -> sprzężenie zwrotne (wzrost prędkości o zadaną wartość)/3(-Fcn(n)), Saturation Dynamic/3
  Saturation Dynamic/1 -> sprzężenie zwrotne (wzrost prędkości o zadaną wartość)/4(y), y/1
  sprzężenie zwrotne (wzrost prędkości o zadaną wartość)/1(sprz) -> IC/1
  u/1 -> sprzężenie zwrotne (wzrost prędkości o zadaną wartość)/2(u), Sum/1
  Sum/1 -> Saturation Dynamic/2
  Fcn/1 -> sprzężenie zwrotne (wzrost prędkości o zadaną wartość)/1(Fcn(n)), Saturation Dynamic/1
  IC/1 -> Sum/2

== system obwod_naprowadzania_JW/MODEL CELU/Model samolotu/Ogranicznik przeciążenia azymut (max 4g) ==
  u : Inport
  v : Inport  Port=2
  Fcn2 : Fcn  Expr=4*9.81/u(1)
  Gain3 : Gain  Gain=-1
  IC : InitialCondition  Value=0
  Saturation Dynamic1 : simulink/Discontinuities/Saturation Dynamic  OutMin=[]  OutMax=[]  OutDataTypeStr=Inherit: Same as second input  OutDataType=fixdt(1, 16)  OutScaling=2^-10  DoSatur=off
  Sum : Sum  Inputs=|++
  sprzężenie zwrotne (skręt o zadany kąt) : Subsystem
  y : Outport
  wires:
  v/1 -> Fcn2/1
  Gain3/1 -> Saturation Dynamic1/3
  Saturation Dynamic1/1 -> sprzężenie zwrotne (skręt o zadany kąt)/3(y), y/1
  Sum/1 -> Saturation Dynamic1/2
  u/1 -> sprzężenie zwrotne (skręt o zadany kąt)/1(u), Sum/1
  Fcn2/1 -> sprzężenie zwrotne (skręt o zadany kąt)/2(Fcn(v)), Saturation Dynamic1/1, Gain3/1
  sprzężenie zwrotne (skręt o zadany kąt)/1(sprz) -> IC/1
  IC/1 -> Sum/2

== system obwod_naprowadzania_JW/MODEL CELU/Model samolotu/Ogranicznik przeciążenia elewacja (max 8g) ==
  u : Inport
  v : Inport  Port=2
  Fcn2 : Fcn  Expr=8*9.81/u(1)
  Gain3 : Gain  Gain=-1
  IC : InitialCondition  Value=0
  Saturation Dynamic1 : simulink/Discontinuities/Saturation Dynamic  OutMin=[]  OutMax=[]  OutDataTypeStr=Inherit: Same as second input  OutDataType=fixdt(1, 16)  OutScaling=2^-10  DoSatur=off
  Sum : Sum  Inputs=|++
  sprzężenie zwrotne (skręt o zadany kąt) : Subsystem
  y : Outport
  wires:
  Gain3/1 -> Saturation Dynamic1/3
  v/1 -> Fcn2/1
  u/1 -> sprzężenie zwrotne (skręt o zadany kąt)/1(u), Sum/1
  Saturation Dynamic1/1 -> sprzężenie zwrotne (skręt o zadany kąt)/3(y), y/1
  Sum/1 -> Saturation Dynamic1/2
  Fcn2/1 -> sprzężenie zwrotne (skręt o zadany kąt)/2(Fcn(v)), Saturation Dynamic1/1, Gain3/1
  sprzężenie zwrotne (skręt o zadany kąt)/1(Out1) -> IC/1
  IC/1 -> Sum/2

== system obwod_naprowadzania_JW/MODEL RAKIETY/10 rownan rozniczkowych/Sub1 ==
  in_1 : Inport
  Fcn : Fcn  Expr=(u[11]*cos(u[17])*cos(u[16])-u[18]-u[12]*g*sin(u[3]))/u[12]
  Integrator : Integrator  InitialCondition=1
  out_1 : Outport
  wires:
  Integrator/1 -> out_1/1
  Fcn/1 -> Integrator/1
  in_1/1 -> Fcn/1

== system obwod_naprowadzania_JW/MODEL RAKIETY/10 rownan rozniczkowych/Sub10 ==
  in_1 : Inport
  Fcn9 : Fcn  Expr=(u[7]*sin(fi)+u[8]*cos(fi))/cos(u[9])
  Integrator9 : Integrator  InitialCondition=atan(y0/x0)+(beta_0_prim_srcp*tster)
  out_1 : Outport
  wires:
  in_1/1 -> Fcn9/1
  Integrator9/1 -> out_1/1
  Fcn9/1 -> Integrator9/1

== system obwod_naprowadzania_JW/MODEL RAKIETY/10 rownan rozniczkowych/Sub2 ==
  in_1 : Inport
  Fcn1 : Fcn  Expr=(u[11]*(sin(u[17])*sin(u[15])+cos(u[17])*sin(u[16])*cos(u[15]))+u[20]*cos(u[15])+u[19]*sin(u[15]))/(u[12]*u[1]*cos(u[3]))
  Integrator1 : Integrator  InitialCondition=atan(y0/x0)+(beta_0_prim_srcp*tster)
  out_1 : Outport
  wires:
  Integrator1/1 -> out_1/1
  Fcn1/1 -> Integrator1/1
  in_1/1 -> Fcn1/1

== system obwod_naprowadzania_JW/MODEL RAKIETY/10 rownan rozniczkowych/Sub3 ==
  in_1 : Inport
  Fcn1 : Fcn  Expr=(u[11]*(sin(u[17])*cos(u[15])+cos(u[17])*sin(u[16])*sin(u[15]))-u[20]*sin(u[15])+u[19]*cos(u[15])-u[12]*g*cos(u[3]))/(u[12]*u[1])
  Integrator3 : Integrator  InitialCondition=(atan(z0/(sqrt(x0^2+y0^2)))+(9.5*pi/180)+(epsilon_0_prim_srcp*tster))*(1/1.05)
  out_1 : Outport
  wires:
  Integrator3/1 -> out_1/1
  in_1/1 -> Fcn1/1
  Fcn1/1 -> Integrator3/1

== system obwod_naprowadzania_JW/MODEL RAKIETY/10 rownan rozniczkowych/Sub4 ==
  in_1 : Inport
  Fcn3 : Fcn  Expr=u[1]*cos(u[3])*cos(u[2])
  Int : Integrator
  out_1 : Outport
  wires:
  in_1/1 -> Fcn3/1
  Int/1 -> out_1/1
  Fcn3/1 -> Int/1

== system obwod_naprowadzania_JW/MODEL RAKIETY/10 rownan rozniczkowych/Sub5 ==
  in_1 : Inport
  Fcn4 : Fcn  Expr=u[1]*cos(u[3])*sin(u[2])
  Integrator4 : Integrator
  out_1 : Outport
  wires:
  in_1/1 -> Fcn4/1
  Integrator4/1 -> out_1/1
  Fcn4/1 -> Integrator4/1

== system obwod_naprowadzania_JW/MODEL RAKIETY/10 rownan rozniczkowych/Sub6 ==
  in_1 : Inport
  Fcn5 : Fcn  Expr=-u[1]*sin(u[3])
  Integrator5 : Integrator
  out_1 : Outport
  wires:
  Integrator5/1 -> out_1/1
  in_1/1 -> Fcn5/1
  Fcn5/1 -> Integrator5/1

== system obwod_naprowadzania_JW/MODEL RAKIETY/10 rownan rozniczkowych/Sub7 ==
  in_1 : Inport
  Fcn6 : Fcn  Expr=u[21]/u[13]
  Integrator6 : Integrator
  out_1 : Outport
  wires:
  Integrator6/1 -> out_1/1
  in_1/1 -> Fcn6/1
  Fcn6/1 -> Integrator6/1

== system obwod_naprowadzania_JW/MODEL RAKIETY/10 rownan rozniczkowych/Sub8 ==
  in_1 : Inport
  Fcn7 : Fcn  Expr=u[22]/u[14]
  Integrator7 : Integrator
  out_1 : Outport
  wires:
  Integrator7/1 -> out_1/1
  in_1/1 -> Fcn7/1
  Fcn7/1 -> Integrator7/1

== system obwod_naprowadzania_JW/MODEL RAKIETY/10 rownan rozniczkowych/Sub9 ==
  in_1 : Inport
  Fcn8 : Fcn  Expr=u[7]*cos(fi)-u[8]*sin(fi)
  Integrator8 : Integrator  InitialCondition=(atan(z0/(sqrt(x0^2+y0^2)))+(9.5*pi/180)+(epsilon_0_prim_srcp*tster))*(1/1.05)
  out_1 : Outport
  wires:
  Integrator8/1 -> out_1/1
  in_1/1 -> Fcn8/1
  Fcn8/1 -> Integrator8/1

== system obwod_naprowadzania_JW/MODEL RAKIETY/Funkcje w rownaniach rozniczkowych/F(t) ==
  in_1 : Inport
  Constant : Constant  Value=ts
  Constant1 : Constant  Value=Fs
  Constant3 : Constant  Value=ts+tm
  Constant4 : Constant  Value=Fm
  Logical Operator : Logic
  Product : Product  InputSameDT=on  RndMeth=Zero  SaturateOnIntegerOverflow=on  OutDataTypeStr=Inherit: Same as first input
  Product1 : Product  InputSameDT=on  RndMeth=Zero  SaturateOnIntegerOverflow=on  OutDataTypeStr=Inherit: Same as first input
  Relational Operator : RelationalOperator  Operator=<=  RndMeth=Nearest  InputSameDT=on
  Relational Operator1 : RelationalOperator  Operator=>  RndMeth=Nearest  InputSameDT=on
  Relational Operator2 : RelationalOperator  Operator=<=  RndMeth=Nearest  InputSameDT=on
  Sum : Sum  InputSameDT=on  SaturateOnIntegerOverflow=on  OutDataTypeStr=Inherit: Same as first input
  out_1 : Outport
  wires:
  in_1/1 -> Relational Operator/1, Relational Operator1/1, Relational Operator2/1
  Constant/1 -> Relational Operator/2, Relational Operator1/2
  Relational Operator/1 -> Product/1
  Constant1/1 -> Product/2
  Product/1 -> Sum/1
  Relational Operator1/1 -> Logical Operator/1
  Relational Operator2/1 -> Logical Operator/2
  Constant3/1 -> Relational Operator2/2
  Logical Operator/1 -> Product1/1
  Constant4/1 -> Product1/2
  Product1/1 -> Sum/2
  Sum/1 -> out_1/1

== system obwod_naprowadzania_JW/MODEL RAKIETY/Funkcje w rownaniach rozniczkowych/Iy(t) Iz(t) ==
  in_1 : Inport
  Constant : Constant  Value=ts
  Constant1 : Constant  Value=Im1
  Constant3 : Constant  Value=ts+tm
  Fcn : Fcn  Expr=((Is1-Is0)/ts)*u(1)+Is0
  Fcn1 : Fcn  Expr=((Im1-Im0)/tm)*u[1]+(ts*(Im0-Im1)+tm*Im0)/tm
  Logical Operator : Logic
  Product : Product  InputSameDT=on  RndMeth=Zero  SaturateOnIntegerOverflow=on  OutDataTypeStr=Inherit: Same as first input
  Product1 : Product  InputSameDT=on  RndMeth=Zero  SaturateOnIntegerOverflow=on  OutDataTypeStr=Inherit: Same as first input
  Product2 : Product  InputSameDT=on  RndMeth=Zero  SaturateOnIntegerOverflow=on  OutDataTypeStr=Inherit: Same as first input
  Relational Operator : RelationalOperator  Operator=<=  RndMeth=Nearest  InputSameDT=on
  Relational Operator1 : RelationalOperator  Operator=>  RndMeth=Nearest  InputSameDT=on
  Relational Operator2 : RelationalOperator  Operator=<=  RndMeth=Nearest  InputSameDT=on
  Relational Operator3 : RelationalOperator  Operator=>  RndMeth=Nearest  InputSameDT=on
  Sum : Sum  Inputs=+++  InputSameDT=on  SaturateOnIntegerOverflow=on  OutDataTypeStr=Inherit: Same as first input
  out_1 : Outport
  wires:
  Constant1/1 -> Product2/2
  Relational Operator3/1 -> Product2/1
  Product1/1 -> Sum/2
  Fcn/1 -> Product/1
  Relational Operator/1 -> Product/2
  in_1/1 -> Fcn/1, Relational Operator/1, Relational Operator3/1, Fcn1/1, Relational Operator2/1, Relational Operator1/1
  Constant/1 -> Relational Operator/2, Relational Operator1/2
  Relational Operator1/1 -> Logical Operator/1
  Relational Operator2/1 -> Logical Operator/2
  Constant3/1 -> Relational Operator3/2, Relational Operator2/2
  Logical Operator/1 -> Product1/1
  Sum/1 -> out_1/1
  Product/1 -> Sum/1
  Product2/1 -> Sum/3
  Fcn1/1 -> Product1/2

== system obwod_naprowadzania_JW/MODEL RAKIETY/Funkcje w rownaniach rozniczkowych/m(t) ==
  in_1 : Inport
  Constant : Constant  Value=ts
  Constant1 : Constant  Value=262.3
  Constant3 : Constant  Value=ts+tm
  Fcn : Fcn  Expr=952.7-(400/ts)*u(1)
  Fcn1 : Fcn  Expr=422.3-(160/tm)*(u(1)-ts)
  Logical Operator : Logic
  Product : Product  InputSameDT=on  RndMeth=Zero  SaturateOnIntegerOverflow=on  OutDataTypeStr=Inherit: Same as first input
  Product1 : Product  InputSameDT=on  RndMeth=Zero  SaturateOnIntegerOverflow=on  OutDataTypeStr=Inherit: Same as first input
  Product2 : Product  InputSameDT=on  RndMeth=Zero  SaturateOnIntegerOverflow=on  OutDataTypeStr=Inherit: Same as first input
  Relational Operator : RelationalOperator  Operator=<=  RndMeth=Nearest  InputSameDT=on
  Relational Operator1 : RelationalOperator  Operator=>  RndMeth=Nearest  InputSameDT=on
  Relational Operator2 : RelationalOperator  Operator=<=  RndMeth=Nearest  InputSameDT=on
  Relational Operator3 : RelationalOperator  Operator=>  RndMeth=Nearest  InputSameDT=on
  Sum : Sum  Inputs=+++  InputSameDT=on  SaturateOnIntegerOverflow=on  OutDataTypeStr=Inherit: Same as first input
  out_1 : Outport
  wires:
  Sum/1 -> out_1/1
  Logical Operator/1 -> Product1/1
  Constant3/1 -> Relational Operator2/2, Relational Operator3/2
  Relational Operator2/1 -> Logical Operator/2
  Relational Operator1/1 -> Logical Operator/1
  Constant/1 -> Relational Operator1/2, Relational Operator/2
  in_1/1 -> Relational Operator1/1, Relational Operator2/1, Fcn1/1, Relational Operator3/1, Relational Operator/1, Fcn/1
  Relational Operator/1 -> Product/2
  Fcn/1 -> Product/1
  Product/1 -> Sum/1
  Fcn1/1 -> Product1/2
  Product1/1 -> Sum/2
  Relational Operator3/1 -> Product2/1
  Constant1/1 -> Product2/2
  Product2/1 -> Sum/3

== system obwod_naprowadzania_JW/MODEL RAKIETY/Zaleznosci na skladowe sil i momentow aerodynamicznych/Cisnienie dynamiczne ==
  In1 : Inport
  In2 : Inport  Port=2
  0.5roV^2 : Product  Inputs=4  InputSameDT=on  RndMeth=Zero  SaturateOnIntegerOverflow=on  OutDataTypeStr=Inherit: Same as first input
  1/2 : Constant  Value=0.5
  Out1 : Outport
  wires:
  1/2/1 -> 0.5roV^2/1
  In1/1 -> 0.5roV^2/2
  0.5roV^2/1 -> Out1/1
  In2/1 -> 0.5roV^2/3, 0.5roV^2/4

== system obwod_naprowadzania_JW/MODEL RAKIETY/Zaleznosci na skladowe sil i momentow aerodynamicznych/PN-78/N-03100   ==
  h : Inport
  cisnienie : Subsystem
  gestosc : Subsystem
  predkosc dzwieku : Subsystem
  temperatura termodynamiczna : Subsystem
  wysokosc geopotencjalna i przyspieszenie : Subsystem
  ro : Outport
  a : Outport  Port=2
  wires:
  h/1 -> wysokosc geopotencjalna i przyspieszenie/1(h)
  wysokosc geopotencjalna i przyspieszenie/1(H) -> cisnienie/1(H), temperatura termodynamiczna/1(H)
  temperatura termodynamiczna/1(T) -> gestosc/2(T), predkosc dzwieku/1(T)
  cisnienie/1(p) -> gestosc/1(p)
  gestosc/1(gestosc) -> ro/1
  predkosc dzwieku/1(predkosc dzwieku) -> a/1

== system obwod_naprowadzania_JW/MODEL RAKIETY/Zaleznosci na skladowe sil i momentow aerodynamicznych/cma ==
  in_1 : Inport
  Constant : Constant
  Fcn : Fcn  Expr=-u(3)*((u(9)-u(10))/caL)*u(1)
  Fcn1 : Fcn  Expr=-u(11)*((u(14)*caL)/u(12))
  Fcn2 : Fcn  Expr=u(4)*((u(10)+0.026745-0.03456*u(13))/caL)*u(7)
  Product : Product  InputSameDT=on  RndMeth=Zero  SaturateOnIntegerOverflow=on  OutDataTypeStr=Inherit: Same as first input
  Sum : Sum  Inputs=+++  InputSameDT=on  SaturateOnIntegerOverflow=on  OutDataTypeStr=Inherit: Same as first input
  out_1 : Outport
  wires:
  in_1/1 -> Fcn/1, Fcn1/1, Fcn2/1
  Fcn1/1 -> Sum/2
  Fcn/1 -> Sum/1
  Fcn2/1 -> Sum/3
  Sum/1 -> Product/1
  Product/1 -> out_1/1
  Constant/1 -> Product/2

== system obwod_naprowadzania_JW/MODEL RAKIETY/Zaleznosci na skladowe sil i momentow aerodynamicznych/cmqa=cnra1 ==
  in_1 : Inport
  Constant : Constant  Value=ts
  Constant2 : Constant  Value=-5.33
  Constant4 : Constant  Value=-0.533
  Product : Product  InputSameDT=on  RndMeth=Zero  SaturateOnIntegerOverflow=on  OutDataTypeStr=Inherit: Same as first input
  Product1 : Product  InputSameDT=on  RndMeth=Zero  SaturateOnIntegerOverflow=on  OutDataTypeStr=Inherit: Same as first input
  Relational Operator : RelationalOperator  Operator=<=  RndMeth=Nearest  InputSameDT=on
  Relational Operator1 : RelationalOperator  Operator=>  RndMeth=Nearest  InputSameDT=on
  Sum : Sum  InputSameDT=on  SaturateOnIntegerOverflow=on  OutDataTypeStr=Inherit: Same as first input
  out_1 : Outport
  wires:
  Product1/1 -> Sum/2
  Constant2/1 -> Product/1
  Relational Operator/1 -> Product/2
  in_1/1 -> Relational Operator/1, Relational Operator1/1
  Constant/1 -> Relational Operator/2, Relational Operator1/2
  Relational Operator1/1 -> Product1/1
  Sum/1 -> out_1/1
  Constant4/1 -> Product1/2
  Product/1 -> Sum/1

== system obwod_naprowadzania_JW/MODEL RAKIETY/Zaleznosci na skladowe sil i momentow aerodynamicznych/cna ==
  in_1 : Inport
  Constant : Constant
  Fcn : Fcn  Expr=u(3)*((u(9)-u(10))/caL)*u(2)
  Fcn1 : Fcn  Expr=-u(11)*((u(15)*caL)/u(12))
  Fcn2 : Fcn  Expr=u(4)*((u(10)+0.026745-0.03456*u(13))/caL)*u(8)
  Product : Product  InputSameDT=on  RndMeth=Zero  SaturateOnIntegerOverflow=on  OutDataTypeStr=Inherit: Same as first input
  Sum : Sum  Inputs=+++  InputSameDT=on  SaturateOnIntegerOverflow=on  OutDataTypeStr=Inherit: Same as first input
  out_1 : Outport
  wires:
  Fcn2/1 -> Sum/3
  Fcn/1 -> Sum/1
  Fcn1/1 -> Sum/2
  in_1/1 -> Fcn2/1, Fcn1/1, Fcn/1
  Sum/1 -> Product/1
  Constant/1 -> Product/2
  Product/1 -> out_1/1

== system obwod_naprowadzania_JW/MODEL RAKIETY/Zaleznosci na skladowe sil i momentow aerodynamicznych/cx ==
  in_1 : Inport
  Fcn : Fcn  Expr=u(5)+u(6)*(u(1)^2+u(2)^2)
  out_1 : Outport
  wires:
  Fcn/1 -> out_1/1
  in_1/1 -> Fcn/1
